simulink model "VectorTrackingSim"  (R2023a)
settings: Solver=FixedStepAuto  StartTime=Start_Time  StopTime=End_Time  FixedStep=Time_Step  RelTol=1e-3
values from neighbouring files (symbols this model uses):
  BSFC_LUT = aircraft.BSFC_LUT    [FVDM_Noise.m]    (also in FVDM_Truth.m)
  STGeometry = aircraft.STGeometry    [FVDM_Noise.m]    (also in FVDM_Truth.m)
  Vehicle = aircraft.Vehicle    [FVDM_Noise.m]    (also in FVDM_Truth.m)
undefined symbols (not defined in the file or in its folder): dayofyear, Earth, Initial_X, lookaheadDist, PowerFactor_LUT, waypoints, WGS84
libraries: slpidlib x7, simulink_extras x3, aerolibtransform2 x1, aerolibatmos2 x1, uavalgslib x1
(part 2 of 2)

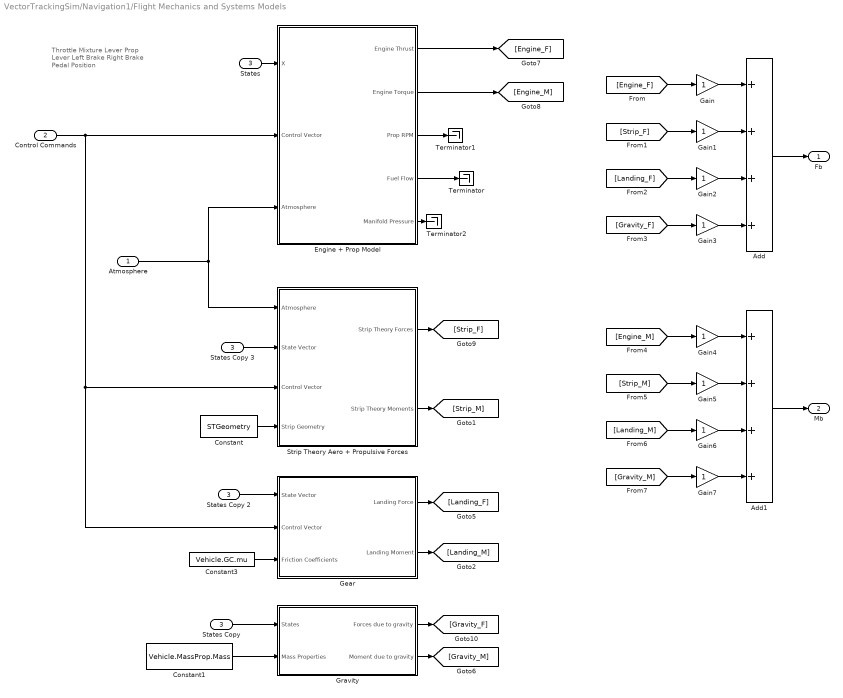
== system VectorTrackingSim/Navigation1/Flight Mechanics and Systems Models ==
  note: Throttle
      | Mixture Lever
      | Prop Lever
      | Left Brake
      | Right Brake
      | Pedal Position
  Atmosphere : Inport
  Control Commands : Inport  Port=2
  States : Inport  Port=3
  Add : Sum  Inputs=++++
  Add1 : Sum  Inputs=++++
  Constant : Constant  Value=STGeometry
  Constant1 : Constant  Value=Vehicle.MassProp.Mass
  Constant3 : Constant  Value=Vehicle.GC.mu
  Engine + Prop Model : Subsystem
  Gain{,1..7} (8 alike) : Gain
  Gear : Subsystem
  Gravity : Subsystem
  States Copy : InportShadow  Port=3
  States Copy 2 : InportShadow  Port=3
  States Copy 3 : InportShadow  Port=3
  Strip Theory Aero + Propulsive Forces : Subsystem
  Terminator : Terminator
  Terminator1 : Terminator
  Terminator2 : Terminator
  Fb : Outport
  Mb : Outport  Port=2
  wires:
  States/1 -> Engine + Prop Model/1(X)
  Constant1/1 -> Gravity/2(Mass Properties)
  Constant/1 -> Strip Theory Aero + Propulsive Forces/4(Strip Geometry)
  Engine + Prop Model/5(Manifold Pressure) -> Terminator2/1
  Engine + Prop Model/3(Prop RPM) -> Terminator1/1
  Constant3/1 -> Gear/3(Friction Coefficients)
  Add1/1 -> Mb/1
  States Copy/1 -> Gravity/1(States)
  States Copy 2/1 -> Gear/1(State Vector)
  States Copy 3/1 -> Strip Theory Aero + Propulsive Forces/2(State Vector)
  Control Commands/1 -> Strip Theory Aero + Propulsive Forces/3(Control Vector), Gear/2(Control Vector), Engine + Prop Model/2(Control Vector)
  Engine + Prop Model/2(Engine Torque) -> [Engine_M]
  Strip Theory Aero + Propulsive Forces/2(Strip Theory Moments) -> [Strip_M]
  Gear/2(Landing Moment) -> [Landing_M]
  Gravity/2(Moment due to gravity) -> [Gravity_M]
  Gravity/1(Forces due to gravity) -> [Gravity_F]
  Gear/1(Landing Force) -> [Landing_F]
  Strip Theory Aero + Propulsive Forces/1(Strip Theory Forces) -> [Strip_F]
  Engine + Prop Model/1(Engine Thrust) -> [Engine_F]
  Add/1 -> Fb/1
  [Engine_F] -> Gain/1
  [Strip_F] -> Gain1/1
  [Landing_F] -> Gain2/1
  [Gravity_F] -> Gain3/1
  [Engine_M] -> Gain4/1
  [Strip_M] -> Gain5/1
  [Landing_M] -> Gain6/1
  [Gravity_M] -> Gain7/1
  Gain/1 -> Add/1
  Gain1/1 -> Add/2
  Gain2/1 -> Add/3
  Gain3/1 -> Add/4
  Gain4/1 -> Add1/1
  Gain5/1 -> Add1/2
  Gain6/1 -> Add1/3
  Gain7/1 -> Add1/4
  Atmosphere/1 -> Strip Theory Aero + Propulsive Forces/1(Atmosphere), Engine + Prop Model/3(Atmosphere)
  Engine + Prop Model/4(Fuel Flow) -> Terminator/1

== system VectorTrackingSim/Guidance/Subsystem/Subsystem1 ==
  Target : Inport
  Demux : Demux  Outputs=3
  Display : Display
  Gain : Gain  Gain=-1
  Terminator : Terminator
  Terminator1 : Terminator
  Altitude : Outport
  wires:
  Target/1 -> Demux/1
  Demux/3 -> Gain/1
  Demux/2 -> Terminator/1
  Demux/1 -> Terminator1/1
  Gain/1 -> Display/1, Altitude/1

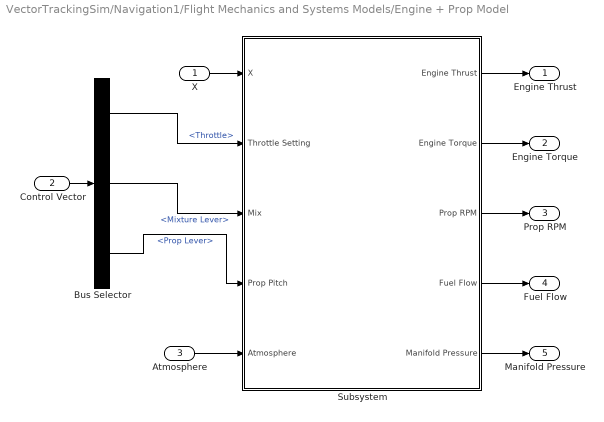
== system VectorTrackingSim/Navigation1/Flight Mechanics and Systems Models/Engine + Prop Model ==
  X : Inport
  Control Vector : Inport  Port=2
  Atmosphere : Inport  Port=3
  Bus Selector : BusSelector  OutputSignals=Throttle,Mixture Lever,Prop Lever
  Subsystem : Subsystem
  Engine Thrust : Outport
  Engine Torque : Outport  Port=2
  Prop RPM : Outport  Port=3  PortDimensions=1
  Fuel Flow : Outport  Port=4  PortDimensions=1
  Manifold Pressure : Outport  Port=5  PortDimensions=1
  wires:
  X/1 -> Subsystem/1(X)
  Subsystem/3(Prop RPM) -> Prop RPM/1
  Subsystem/4(Fuel Flow) -> Fuel Flow/1
  Subsystem/5(Manifold Pressure) -> Manifold Pressure/1
  Control Vector/1 -> Bus Selector/1
  Bus Selector/1 -> Subsystem/2(Throttle Setting)  "<Throttle>"
  Bus Selector/2 -> Subsystem/3(Mix)  "<Mixture Lever>"
  Bus Selector/3 -> Subsystem/4(Prop Pitch)  "<Prop Lever>"
  Atmosphere/1 -> Subsystem/5(Atmosphere)
  Subsystem/2(Engine Torque) -> Engine Torque/1
  Subsystem/1(Engine Thrust) -> Engine Thrust/1

== system VectorTrackingSim/Navigation1/Flight Mechanics and Systems Models/Gear ==
  State Vector : Inport
  Control Vector : Inport  Port=2
  Friction Coefficients : Inport  Port=3
  " " : MATLAB Function  TreatAsAtomicUnit=on
  Bus Selector : BusSelector  OutputSignals=LeftBrake,RightBrake,Pedal Posn
  Mux : Mux  Inputs=3
  Landing Force : Outport
  Landing Moment : Outport  Port=2
  wires:
  Friction Coefficients/1 -> " "/3(mu)
  State Vector/1 -> " "/2(X)
  " "/1(Ground_Forces) -> Landing Force/1
  " "/2(Ground_Moments) -> Landing Moment/1
  Control Vector/1 -> Bus Selector/1
  Mux/1 -> " "/1(U)
  Bus Selector/1 -> Mux/1  "<LeftBrake>"
  Bus Selector/2 -> Mux/2  "<RightBrake>"
  Bus Selector/3 -> Mux/3  "<Pedal Posn>"

== system VectorTrackingSim/Navigation1/Flight Mechanics and Systems Models/Gravity ==
  States : Inport
  Mass Properties : Inport  Port=2
  Constant : Constant  Value=Vehicle.MassProp.r_cg
  MATLAB Function : MATLAB Function  TreatAsAtomicUnit=on
  Forces due to gravity : Outport
  Moment due to gravity : Outport  Port=2
  wires:
  MATLAB Function/1(F_grav_b) -> Forces due to gravity/1
  States/1 -> MATLAB Function/1(X)
  Mass Properties/1 -> MATLAB Function/2(Mass_Properties)
  MATLAB Function/2(M_grav_b) -> Moment due to gravity/1
  Constant/1 -> MATLAB Function/3(CG)

== system VectorTrackingSim/Navigation1/Flight Mechanics and Systems Models/Strip Theory Aero + Propulsive Forces ==
  Atmosphere : Inport
  State Vector : Inport  Port=2
  Control Vector : Inport  Port=3
  Strip Geometry : Inport  Port=4
  Strip_Theory_Modeling : MATLAB Function  TreatAsAtomicUnit=on
  Strip Theory Forces : Outport
  Strip Theory Moments : Outport  Port=2
  wires:
  Atmosphere/1 -> Strip_Theory_Modeling/1(atmos)
  Strip Geometry/1 -> Strip_Theory_Modeling/4(stripGeom)
  Control Vector/1 -> Strip_Theory_Modeling/3(U)
  State Vector/1 -> Strip_Theory_Modeling/2(X)
  Strip_Theory_Modeling/1(Strip_Theory_Forces) -> Strip Theory Forces/1
  Strip_Theory_Modeling/2(Strip_Theory_Moments) -> Strip Theory Moments/1

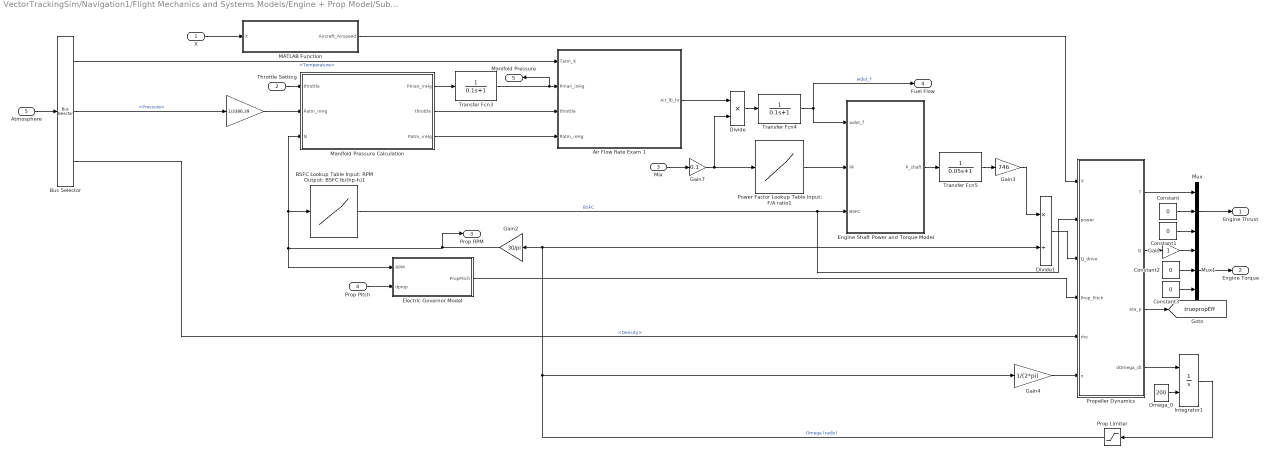
== system VectorTrackingSim/Navigation1/Flight Mechanics and Systems Models/Engine + Prop Model/Subsystem ==
  X : Inport
  Throttle Setting : Inport  Port=2
  Mix : Inport  Port=3
  Prop Pitch : Inport  Port=4
  Atmosphere : Inport  Port=5
  " " : Gain  Gain=1/3386.39
  Air Flow Rate Exam 1 : MATLAB Function  TreatAsAtomicUnit=on
  BSFC Lookup Table Input: RPM Output: BSFC lb/(hp-h)1 : Lookup_n-D  NumberOfTableDimensions=1  BreakpointsForDimension1=BSFC_LUT(1,:)  Table=BSFC_LUT(2,:)  ExtrapMethod=Clip  UseLastTableValue=on  InternalRulePriority=Speed  RndMeth=Simplest
  Bus Selector : BusSelector  OutputSignals=Temperature,Pressure,Density
  Constant{,1..3} (4 alike) : Constant  Value=0
  Divide : Product  Inputs=**
  Divide1 : Product  Inputs=*/
  Electric Governor Model : Subsystem
  Engine Shaft Power and Torque Model : MATLAB Function  TreatAsAtomicUnit=on
  Gain : Gain
  Gain2 : Gain  Gain=30/pi
  Gain3 : Gain  Gain=746
  Gain4 : Gain  Gain=1/(2*pi)
  Gain7 : Gain  Gain=0.1
  Integrator1 : Integrator  InitialConditionSource=external
  MATLAB Function : MATLAB Function  TreatAsAtomicUnit=on
  Manifold Pressure Calculation : MATLAB Function  TreatAsAtomicUnit=on
  Mux : Mux  Inputs=3
  Mux1 : Mux  Inputs=3
  Omega_0 : Constant  Value=200
  Power Factor Lookup Table Input: F/A ratio1 : Lookup_n-D  NumberOfTableDimensions=1  BreakpointsForDimension1=PowerFactor_LUT(1,:)  Table=PowerFactor_LUT(2,:)  ExtrapMethod=Clip  UseLastTableValue=on  InternalRulePriority=Speed  RndMeth=Simplest
  Prop Limiter : Saturate  UpperLimit=320  LowerLimit=0
  Propeller Dynamics : MATLAB Function  TreatAsAtomicUnit=on
  Transfer Fcn3 : TransferFcn  Denominator=[0.1 1]
  Transfer Fcn4 : TransferFcn  Denominator=[0.1 1]
  Transfer Fcn5 : TransferFcn  Denominator=[0.05 1]
  Engine Thrust : Outport
  Engine Torque : Outport  Port=2
  Prop RPM : Outport  Port=3  PortDimensions=1
  Fuel Flow : Outport  Port=4  PortDimensions=1
  Manifold Pressure : Outport  Port=5  PortDimensions=1
  tag scope: truepropEff=global
  wires:
  Transfer Fcn4/1 -> Engine Shaft Power and Torque Model/1(wdot_f), Fuel Flow/1  "wdot_f"
  Constant2/1 -> Mux1/2
  Propeller Dynamics/4(dOmega_dt) -> Integrator1/1
  Mux/1 -> Engine Thrust/1
  Gain2/1 -> Prop RPM/1, Electric Governor Model/1(RPM), BSFC Lookup Table Input: RPM Output: BSFC lb/(hp-h)1/1, Manifold Pressure Calculation/3(N)
  Electric Governor Model/1(PropPitch) -> Propeller Dynamics/4(Prop_Pitch)
  Divide/1 -> Transfer Fcn4/1
  Propeller Dynamics/3(eta_p) -> [truepropEff]
  Constant/1 -> Mux/2
  Gain4/1 -> Propeller Dynamics/6(n)
  Mix/1 -> Gain7/1
  Bus Selector/3 -> Propeller Dynamics/5(rho)  "<Density>"
  Manifold Pressure Calculation/3(Patm_inHg) -> Air Flow Rate Exam 1/4(Patm_inHg)
  BSFC Lookup Table Input: RPM Output: BSFC lb/(hp-h)1/1 -> Propeller Dynamics/2(power), Engine Shaft Power and Torque Model/3(BSFC)  "BSFC"
  Manifold Pressure Calculation/2(throttle) -> Air Flow Rate Exam 1/3(throttle)
  Prop Limiter/1 -> Divide1/2, Gain2/1, Gain4/1  "Omega (rad/s)"
  Propeller Dynamics/1(T) -> Mux/1
  Engine Shaft Power and Torque Model/1(P_shaft) -> Transfer Fcn5/1
  Omega_0/1 -> Integrator1/2
  Constant3/1 -> Mux1/3
  Transfer Fcn3/1 -> Manifold Pressure/1, Air Flow Rate Exam 1/2(Pman_inHg)
  Power Factor Lookup Table Input: F/A ratio1/1 -> Engine Shaft Power and Torque Model/2(PF)
  X/1 -> MATLAB Function/1(X)
  Gain3/1 -> Divide1/1
  Prop Pitch/1 -> Electric Governor Model/2(dprop)
  Transfer Fcn5/1 -> Gain3/1
  Propeller Dynamics/2(Q) -> Gain/1
  Mux1/1 -> Engine Torque/1
  Gain/1 -> Mux1/1
  Divide1/1 -> Propeller Dynamics/3(Q_drive)
  Manifold Pressure Calculation/1(Pman_inHg) -> Transfer Fcn3/1
  Gain7/1 -> Power Factor Lookup Table Input: F/A ratio1/1, Divide/2
  MATLAB Function/1(Aircraft_Airspeed) -> Propeller Dynamics/1(V)
  Throttle Setting/1 -> Manifold Pressure Calculation/1("throttle ")
  " "/1 -> Manifold Pressure Calculation/2("Patm_inHg ")
  Constant1/1 -> Mux/3
  Atmosphere/1 -> Bus Selector/1
  Bus Selector/1 -> Air Flow Rate Exam 1/1(Tatm_K)  "<Temperature>"
  Bus Selector/2 -> " "/1  "<Pressure>"
  Air Flow Rate Exam 1/1(Air_lb_hr) -> Divide/1
  Integrator1/1 -> Prop Limiter/1

== system VectorTrackingSim/Navigation1/Flight Mechanics and Systems Models/Engine + Prop Model/Subsystem/Electric Governor Model ==
  RPM : Inport
  dprop : Inport  Port=2
  Constant : Constant  Value=0
  DESIRED RPM : MATLABFcn  MATLABFcn=800 + 2000 * u
  Initial Blade Pitch : Constant  Value=5
  PID Controller (2DOF) : slpidlib/PID Controller (2DOF)  Controller=PID  Form=Parallel  TimeDomain=Continuous-time  UseExternalTs=off  SampleTime=-1  IntegratorMethod=Forward Euler  FilterMethod=Forward Euler  ControllerParametersSource=internal  P=-.08  I=-0.01  UseKiTs=off  D=0  N=100  UseFilter=on  b=1  c=0  TunerSelectOption=Transfer Function Based (PID Tuner App)  InitialConditionSource=external  InitialConditionForIntegrator=0  InitialConditionForFilter=0  DifferentiatorICPrevScaledInput=0  ExternalReset=none  TrackingMode=off  Kt=1  LimitOutput=on  SatLimitsSource=internal  UpperSaturationLimit=26  LowerSaturationLimit=10  LinearizeAsGain=on  AntiWindupMode=clamping  Kb=1  LimitIntegrator=off  UpperIntegratorSaturationLimit=inf  LowerIntegratorSaturationLimit=-inf  POutMin=[]  POutMax=[]  IOutMin=[]  IOutMax=[]  DOutMin=[]  DOutMax=[]  NOutMin=[]  NOutMax=[]  bOutMin=[]  bOutMax=[]  cOutMin=[]  cOutMax=[]  SumOutMin=[]  SumOutMax=[]  SaturationOutMin=[]  SaturationOutMax=[]  PParamMin=[]  PParamMax=[]  IParamMin=[]  IParamMax=[]  DParamMin=[]  DParamMax=[]  NParamMin=[]  NParamMax=[]  bParamMin=[]  bParamMax=[]  cParamMin=[]  cParamMax=[]  KbParamMin=[]  KbParamMax=[]  KtParamMin=[]  KtParamMax=[]  KbOutMin=[]  KbOutMax=[]  KtOutMin=[]  KtOutMax=[]  IntegratorOutMin=[]  IntegratorOutMax=[]  FilterOutMin=[]  FilterOutMax=[]  SumI1OutMin=[]  SumI1OutMax=[]  SumI2OutMin=[]  SumI2OutMax=[]  SumI3OutMin=[]  SumI3OutMax=[]  SumI4OutMin=[]  SumI4OutMax=[]  SumDOutMin=[]  SumDOutMax=[]  Sum1OutMin=[]  Sum1OutMax=[]  Sum2OutMin=[]  Sum2OutMax=[]  Sum3OutMin=[]  Sum3OutMax=[]  DifferentiatorOutMin=[]  DifferentiatorOutMax=[]  FilterDiffOutCoefMin=[]  FilterDiffOutCoefMax=[]  ReciprocalOutMin=[]  ReciprocalOutMax=[]  SumDenOutMin=[]  SumDenOutMax=[]  SumNumOutMin=[]  SumNumOutMax=[]  DivideOutMin=[]  DivideOutMax=[]  UdiffTsProdOutMin=[]  UdiffTsProdOutMax=[]  NTsProdOutMin=[]  NTsProdOutMax=[]  UintegralTsProdOutMin=[]  UintegralTsProdOutMax=[]  UngainTsProdOutMin=[]  UngainTsProdOutMax=[]  ClampingZeroOutDataTypeStr=Inherit: Inherit via back propagation  ClampingZeroOutMin=[]  ClampingZeroOutMax=[]  FilterDenConstantOutDataTypeStr=Inherit: Inherit via back propagation  FilterDenConstantOutMin=[]  FilterDenConstantOutMax=[]  PCopyOutDataTypeStr=Inherit: Inherit via back propagation  PCopyOutMin=[]  PCopyOutMax=[]  NCopyOutDataTypeStr=Inherit: Inherit via back propagation  NCopyOutMin=[]  NCopyOutMax=[]  IntegratorContinuousStateAttributes=''  IntegratorStateMustResolveToSignalObject=off  IntegratorRTWStateStorageClass=Auto  FilterContinuousStateAttributes=''  FilterStateMustResolveToSignalObject=off  FilterRTWStateStorageClass=Auto  ParallelPVariant=InternalParameters  IdealPVariant=Disabled  IVariant=InternalParameters  DVariant=InternalParameters  bVariant=InternalParameters  cVariant=InternalParameters  IntegratorVariant=Continuous  SatVariant=Enabled  AWVariant=ContClampingParallel  PCopyVariant=Disabled  TRVariant=Disabled  FdbkBlocksVariant=Forward  IdealPFdbkVariant=Disabled  SatFdbkVariant=Disabled  DerivativeFilterVariant=ContFilter  NVariant=InternalParameters  NCopyVariant=Disabled  FilterICVariant=ExternalICs  IntegratorICVariant=ExternalICs  ExternalResetVariant=Disabled  TRSumVariant=Passthrough  SumFdbkVariant=Disabled  SumVariant=Sum_PID  TsampFilterVariant=InternalTs  TsampNgainVariant=Passthrough  TsampIntegralVariant=Disabled_SignalSpec  ExternalSaturationOutDataTypeStr=Inherit: Same as second input
  Saturation : Saturate  UpperLimit=2650  LowerLimit=800
  PropPitch : Outport
  wires:
  dprop/1 -> DESIRED RPM/1
  PID Controller (2DOF)/1 -> PropPitch/1
  Constant/1 -> PID Controller (2DOF)/4
  Initial Blade Pitch/1 -> PID Controller (2DOF)/3
  DESIRED RPM/1 -> Saturation/1
  RPM/1 -> PID Controller (2DOF)/2
  Saturation/1 -> PID Controller (2DOF)/1

== matlab function VectorTrackingSim/Navigation1/Flight Mechanics and Systems Models/Engine + Prop Model/Subsystem/Propeller Dynamics ==
  data: V input; power input; Q_drive input size=1; Prop_Pitch input; rho input; n input; T output; Q output; eta_p output size=1; dOmega_dt output
function [T,Q,eta_p,dOmega_dt] = VarP_PropDynamics(V,power, Q_drive,Prop_Pitch,rho,n)

T = 0;
Q = 0;
eta_p = 0;
dOmega_dt = 0;

coder.extrinsic('griddedInterpolant')
coder.extrinsic('CTCQPropeff')

[T,Q,eta_p,dOmega_dt] = CTCQPropeff(Prop_Pitch,power,Q_drive,rho,V,n,[]);

end

== matlab function VectorTrackingSim/Navigation1/Flight Mechanics and Systems Models/Gear/  ==
  data: U input; X input; mu input; Ground_Forces output; Ground_Moments output
function [Ground_Forces,Ground_Moments] = LDG_Model(U,X,mu)
%% Ground Contact points taken from powerpoint
Front_LDG = [1.634;0;0.983]';
Right_MG = [-0.5;1.447;0.893]';
Left_MG = [-0.5;-1.447;0.893]';
Prop_Strike = [2.379;0;0.847]';
Right_Wing = [0;5.53;-0.087]';
Left_Wing = [0;-5.53;-0.087]';
Tail_Strike = [-4.552;0;0.271]';
GC = [Front_LDG;Right_MG;Left_MG;Prop_Strike;Right_Wing;Left_Wing;Tail_Strike];
%% Spring and Damper Coeffs
k_r = 80000;
c_r = 14300;

k_f = 50000;
c_f = 11300;

k_b = 280000;
c_b = 26800;
%% Defining State Vector to make the coding easier
u = X(1);
v = X(2);
w = X(3);
p = X(4);
q = X(5);
r = X(6);
x = X(7);
y = X(8);
z = X(9);
phi = X(10);
theta = X(11);
psi = X(12);

ALTdot = -w;
ALT = -z;
%% State Derivatives
phidot = p + q*sin(phi)*tan(theta) + r*cos(phi)*tan(theta);
thetadot = q*cos(phi) - r*sin(phi);
%% Controls from Pilot
Brake_Setting = (U(1) + U(2))/2;
Steering_Control = U(3);
%% Friction while plane is in motion
Rolling_Friction = mu(1);
%% Calculations
%% Have to calculate each components distance from the ground...
del_S = zeros(7,1);
del_S_dot = zeros(7,1);
F = zeros(7,3);

del_S(1) = ALT + Front_LDG(1)*sin(theta) - Front_LDG(2)*sin(phi)*cos(theta) - Front_LDG(3)*cos(phi)*cos(theta);
del_S(2) = ALT + Right_MG(1)*sin(theta) - Right_MG(2)*sin(phi)*cos(theta) - Right_MG(3)*cos(phi)*cos(theta);
del_S(3) = ALT + Left_MG(1)*sin(theta) - Left_MG(2)*sin(phi)*cos(theta) - Left_MG(3)*cos(phi)*cos(theta);
del_S(4) = ALT + Prop_Strike(1)*sin(theta) - Prop_Strike(2)*sin(phi)*cos(theta) - Prop_Strike(3)*cos(phi)*cos(theta);
del_S(5) = ALT + Right_Wing(1)*sin(theta) - Right_Wing(2)*sin(phi)*cos(theta) - Right_Wing(3)*cos(phi)*cos(theta);
del_S(6) = ALT + Left_Wing(1)*sin(theta) - Left_Wing(2)*sin(phi)*cos(theta) - Left_Wing(3)*cos(phi)*cos(theta);
del_S(7) = ALT + Tail_Strike(1)*sin(theta) - Tail_Strike(2)*sin(phi)*cos(theta) - Tail_Strike(3)*cos(phi)*cos(theta);

%deltaS order
% 1 Nose Gear
% 2 Right Main Gear
% 3 Left Main Gear
% 4 Prop Strike
% 5 Right Wingtip
% 6 Left Wingtip
% 7 Tail Strike

del_S_dot(1) = ALTdot + Front_LDG(1)*cos(theta)*thetadot + Front_LDG(2)*(thetadot*sin(phi)*sin(theta) - phidot*cos(phi)*cos(theta)) + Front_LDG(3)*(thetadot*sin(theta)*cos(phi) + phidot*sin(theta)*sin(phi))+ del_S(1)*(cos(phi)*sin(theta)*thetadot + sin(phi)*cos(theta)*phidot);
if del_S(1) < 0
    F(1,3) = k_f*del_S(1) + c_f*del_S_dot(1);
else
    F(1,3) = 0;
end
del_S_dot(2) = ALTdot + Right_MG(1)*cos(theta)*thetadot + Right_MG(2)*(thetadot*sin(phi)*sin(theta) - phidot*cos(phi)*cos(theta)) + Right_MG(3)*(thetadot*sin(theta)*cos(phi) + phidot*sin(theta)*sin(phi))+ del_S(2)*(cos(phi)*sin(theta)*thetadot + sin(phi)*cos(theta)*phidot);
if del_S(2) < 0
    F(2,3) = k_r*del_S(2) + c_r*del_S_dot(2);
else
    F(2,3) = 0;
end
del_S_dot(3) = ALTdot + Left_MG(1)*cos(theta)*thetadot + Left_MG(2)*(thetadot*sin(phi)*sin(theta) - phidot*cos(phi)*cos(theta)) + Left_MG(3)*(thetadot*sin(theta)*cos(phi) + phidot*sin(theta)*sin(phi))+ del_S(3)*(cos(phi)*sin(theta)*thetadot + sin(phi)*cos(theta)*phidot);
if del_S(3) < 0
    F(3,3) = k_r*del_S(3) + c_r*del_S_dot(3);
else
    F(3,3) = 0;
end
del_S_dot(4) = ALTdot + Prop_Strike(1)*cos(theta)*thetadot + Prop_Strike(2)*(thetadot*sin(phi)*sin(theta) - phidot*cos(phi)*cos(theta)) + Prop_Strike(3)*(thetadot*sin(theta)*cos(phi) + phidot*sin(theta)*sin(phi));
if del_S(4) < 0
    F(4,3) = k_b*del_S(4) + c_b*del_S_dot(4);
else
    F(4,3) = 0;
end
del_S_dot(5) = ALTdot + Right_Wing(1)*cos(theta)*thetadot + Right_Wing(2)*(thetadot*sin(phi)*sin(theta) - phidot*cos(phi)*cos(theta)) + Right_Wing(3)*(thetadot*sin(theta)*cos(phi) + phidot*sin(theta)*sin(phi));
if del_S(5) < 0
    F(5,3) = k_b*del_S(5) + c_b*del_S_dot(5);
else
    F(5,3) = 0;
end
del_S_dot(6) = ALTdot + Left_Wing(1)*cos(theta)*thetadot + Left_Wing(2)*(thetadot*sin(phi)*sin(theta) - phidot*cos(phi)*cos(theta))+ Left_Wing(3)*(thetadot*sin(theta)*cos(phi) + phidot*sin(theta)*sin(phi));
if del_S(6) < 0
    F(6,3) = k_b*del_S(6) + c_b*del_S_dot(6);
else
    F(6,3) = 0;
end

del_S_dot(7) = ALTdot + Tail_Strike(1)*cos(theta)*thetadot + Tail_Strike(2)*(thetadot*sin(phi)*sin(theta) - phidot*cos(phi)*cos(theta)) + Tail_Strike(3)*(thetadot*sin(theta)*cos(phi) + phidot*sin(theta)*sin(phi));
if del_S(7) < 0
    F(7,3) = k_b*del_S(7) + c_b*del_S_dot(7);
else
    F(7,3) = 0;
end
%% Calculating the velo seen by the LDG

VxB = u - r.*GC(:,2) + q.*(GC(:,3) + del_S);
VyB = v + r.*GC(:,1) - p.*(GC(:,3) + del_S);
VzB = w - q.*GC(:,1) + p.*GC(:,2);

Vxge = cos(theta).*VxB + (sin(phi).*sin(theta)).*VyB + (cos(phi)*sin(theta)).*VzB;
Vyge = cos(phi).*VyB + (-sin(phi)).*VzB;

Steering_Control = [Steering_Control,0,0,0,0,0,0]';
uk  = VxB.*cos(Steering_Control) + VyB.*sin(Steering_Control);

mu_s = 0.8;
C_p = 1.1;
B_p = 7;
mu_br = 0.7*Brake_Setting;
mu_rb = zeros(3,1);
mu_Y = zeros(3,1);
for i = 1:3
    if abs(uk(i)) < 1e-4
        mu_rb(i) = 0;
    else
        mu_rb(i) =  (Rolling_Friction + mu_br).*sign(uk(i));
    end
    
    mu_y_max = sqrt(mu_s^2 - mu_rb(i)^2);
    Sy =  Steering_Control(i) - atan(Vyge(i)/(Vxge(i) + 0.00000001 ));
    if abs(uk(i)) < 0.001
        mu_Y(i) = 0;
    else
        mu_Y(i) = -mu_y_max*sin(C_p*atan(B_p.*Sy));
    end
end
%% Calculating the x and y forces...
F(1:3,1) = mu_rb.*F(1:3,3);
F(1:3,2) = mu_Y.*F(1:3,3);
%% Converting to Body-Fixed Axis to output...
F_B = zeros(7,3);
F_B(:,1) = cos(theta).*cos(-Steering_Control).*F(:,1) + cos(theta).*F(:,2) - sin(theta).*F(:,3);
F_B(:,2)= (sin(phi).*sin(theta).*cos(-Steering_Control)-cos(phi).*sin(-Steering_Control)).*F(:,1) + (sin(phi).*sin(theta).*sin(-Steering_Control) + cos(phi).*cos(-Steering_Control)).*F(:,2) + sin(phi).*cos(theta).*F(:,3);
F_B(:,3) = (cos(phi).*sin(theta).*cos(-Steering_Control) + sin(phi).*sin(-Steering_Control)).*F(:,1) + (cos(phi).*sin(theta).*sin(-Steering_Control)-sin(phi).*cos(-Steering_Control)).*F(:,2) + (cos(phi).*cos(theta)).*F(:,3);

NG_Mom = cross(Front_LDG,F(1,:));
RMG_Mom = cross(Right_MG, F(2,:));
LMG_Mom = cross(Left_MG, F(3,:));
Prop_Strike_Mom = cross(Prop_Strike,F(4,:));
RWT_Mom = cross(Right_Wing,F(5,:));
LWT_Mom = cross(Left_Wing,F(6,:));
Tail_Strike_Mom = cross(Tail_Strike, F(7,:));

Ground_Forces = [sum(F_B(:,1)),sum(F_B(:,2)),sum(F_B(:,3))];
Ground_Moments = (NG_Mom + RMG_Mom + LMG_Mom + Prop_Strike_Mom + RWT_Mom + LWT_Mom + Tail_Strike_Mom);
end

== matlab function VectorTrackingSim/Navigation1/Flight Mechanics and Systems Models/Gravity/MATLAB Function ==
  data: X input; F_grav_b output; Mass_Properties input; CG input; M_grav_b output
function [F_grav_b,M_grav_b] = Grav_Forces(X,Mass_Properties,CG)
%% Defining State Vector to Code Easier
u = X(1);
v = X(2);
w = X(3);
p = X(4);
q = X(5);
r = X(6);
x = X(7);
y = X(8);
z = X(9);
phi = X(10);
theta = X(11);
psi = X(12);

g = 9.81;

F_grav_b = Mass_Properties.*[-g*sin(theta);g*sin(phi)*cos(theta);g*cos(phi)*cos(theta)];

M_grav_b = cross(CG,F_grav_b);

== matlab function VectorTrackingSim/Navigation1/Flight Mechanics and Systems Models/Strip Theory Aero + Propulsive Forces/Strip_Theory_Modeling ==
  data: atmos input; X input; U input; stripGeom input; Strip_Theory_Forces output; Strip_Theory_Moments output
function [Strip_Theory_Forces,Strip_Theory_Moments] = Strip_Theory(atmos,X,U,stripGeom)
Strip_Theory_Forces = [0;0;0];
Strip_Theory_Moments = [0;0;0];

coder.extrinsic('griddedInterpolant')
coder.extrinsic('AC_Strip_Theory')

[Strip_Theory_Forces,Strip_Theory_Moments] = AC_Strip_Theory(atmos(4),X,U,stripGeom);

== matlab function VectorTrackingSim/Control/Subsystem3/MATLAB Function ==
  data: X input; Aircraft_Airspeed output
function Aircraft_Airspeed = Calc_AC_Speed(X)
Aircraft_Airspeed = norm(X(1:3));
end

== matlab function VectorTrackingSim/Navigation1/DA-40 Equations of Motion/MATLAB Function4 ==
  data: m input; X_Dot output size=12; Ic_B input; F_B input; M_B input; X input; CG input; InvMassMatrix input
function X_Dot  = CalcXdot(m,Ic_B,F_B,M_B,X,CG,InvMassMatrix)
X_Dot = zeros(12,1);
% muVector = zeros(3,1);
u = X(1);
v = X(2);
w = X(3);
p = X(4);
q = X(5);
r = X(6);
x = X(7);
y = X(8);
z = X(9);
phi = X(10);
theta = X(11);
psi = X(12);


Xcg = CG(1);
Ycg = CG(2);
Zcg = CG(3);

CGssm = [0 -Zcg Ycg;Zcg 0 -Xcg;-Ycg Xcg 0];


lambdaX = F_B(1)/m + r*v - q*w - 0 - 2*q*0 + 2*r*0 + Xcg*(q^2 + r^2) - Ycg*p*q - Zcg*p*r;
lambdaY = F_B(2)/m + p*w - r*u - 0 - 2*r*0 + 2*p*0 - Xcg*p*q + Ycg*(p^2 +r^2) - Zcg*q*r;
lambdaZ = F_B(3)/m + q*u - p*v - 0 - 2*p*0 + 2*q*0 - Xcg*p*r - Ycg*q*r + Zcg*(p^2 + q^2);

MomentVector = [p;q;r];

MomentVectorssm = [0 -r q;r 0 -p;-q p 0];

muVector = [M_B(1);M_B(2);M_B(3)] - (MomentVectorssm*Ic_B*MomentVector) - m*CGssm*MomentVectorssm*[u;v;w];
LAMEparams = [lambdaX;lambdaY;lambdaZ;muVector];
X_Dot(1:6) = InvMassMatrix*LAMEparams;

cphi = cos(phi);
sphi = sin(phi);

ctheta = cos(theta);
stheta = sin(theta);
ttheta = tan(theta);

cpsi = cos(psi);
spsi = sin(psi);

xdot = ctheta*cpsi*u + sphi*stheta*cpsi - cphi*spsi*v + cphi*stheta*cpsi + sphi*spsi*w;
ydot = ctheta*spsi*u + sphi*stheta*spsi + cphi*cpsi*v + cphi*stheta*spsi - sphi*cpsi*w;
zdot = -stheta*u + sphi*ctheta*v + cphi*ctheta*w;
phidot = p + q*sphi*ttheta + r*cphi*ttheta;
thdot = q*cphi - r*sphi;
psidot = q*sphi/ctheta + r*cphi/ctheta;
X_Dot(7:12) = [xdot;ydot;zdot;phidot;thdot;psidot];

end

== matlab function VectorTrackingSim/Guidance/MATLAB Function ==
  data: heading input; heading output
function heading = fcn(heading)

heading = wrapTo360(heading*180/pi);

end

== matlab function VectorTrackingSim/Environment/MATLAB Function ==
  data: windVectorNav input; windVectorBody output; states input
function windVectorBody = windRotation(windVectorNav,states)

DCMBN = genDCM('rad',[states(12),states(11),states(10)], [3 2 1]);

windVectorBody = DCMBN'*[windVectorNav; 0];

end

== matlab function VectorTrackingSim/Navigation1/Flight Mechanics and Systems Models/Engine + Prop Model/Subsystem/Air Flow Rate Exam 1 ==
  data: Tatm_K input; Pman_inHg input; throttle input; Patm_inHg input; Air_lb_hr output
function Air_lb_hr  = Calc_Air_Flow(Tatm_K,Pman_inHg,throttle,Patm_inHg)
%% Conversion Factors
inHg_to_Pa = 3386.39;
in2_to_m2 = 0.00064516;
kg_to_lb = 2.20462;
%% Constants
gamma = 1.4;
R = 287;
AirflowScaler = 0.69 * 0.95;
DischargeCoeff = 0.6;
th = 70*throttle;
D = 2.75;

Patm_Pa = Patm_inHg * inHg_to_Pa;
Pman_Pa = Pman_inHg * inHg_to_Pa;
A_in2 = (pi/4) * D^2 *  (0.01 + (1-0.01)*(1 - cosd(th)));
A_m2 = A_in2 * in2_to_m2;

Threshold_X = (2/(gamma+1))^(gamma/(gamma-1));

x = Threshold_X;

MAF = sqrt((2*gamma/(gamma-1))*(x^(2/gamma)-x^((gamma+1)/gamma)));

MassFlux_kgm2s = MAF*Patm_Pa/sqrt(R*Tatm_K);
MassFlow_kgs = MassFlux_kgm2s * A_m2; 

Air_lb_hr = AirflowScaler*DischargeCoeff*MassFlow_kgs*3600*kg_to_lb;
end

== matlab function VectorTrackingSim/Navigation1/Flight Mechanics and Systems Models/Engine + Prop Model/Subsystem/Engine Shaft Power and Torque Model ==
  data: wdot_f input; PF input; BSFC input; P_shaft output
function P_shaft  = fcn(wdot_f,PF,BSFC)

P_shaft = PF*wdot_f/BSFC; %hp

% Q_drive = P_shaft*746/Omega; %Nm


end

== matlab function VectorTrackingSim/Navigation1/Flight Mechanics and Systems Models/Engine + Prop Model/Subsystem/MATLAB Function ==
  data: X input; Aircraft_Airspeed output
function Aircraft_Airspeed = Calc_AC_Speed(X)
Aircraft_Airspeed = norm(X(1:3));
end

== matlab function VectorTrackingSim/Navigation1/Flight Mechanics and Systems Models/Engine + Prop Model/Subsystem/Manifold Pressure Calculation ==
  data: throttle input; Patm_inHg input; N input; Pman_inHg output; throttle output; Patm_inHg output
function [Pman_inHg,throttle,Patm_inHg]  = fcn(throttle,Patm_inHg,N)

Pman_inHg = Patm_inHg + (0.007*throttle - 0.0086)*N;

end
